simulink model "sldemo_msfcn_edge_detect"  (Simulink 7.6)
settings: Solver=ode45  StartTime=0.0  StopTime=inf  RelTol=1e-3
settings Model: Creator=The MathWorks Inc.  ExtModeAutoUpdateStatusClock=off
settings DataIOCC: SignalLoggingName=logsOut
settings OptimizationCC: InlineInvariantSignals=on  InitFltsAndDblsToZero=on
settings DebuggingCC: SaveWithParameterizedLinksMsg=none  SignalResolutionControl=TryResolveAllWithWarning  SolverPrmCheckMsg=none  InheritedTsInSrcMsg=none  MultiTaskDSMMsg=warning  MultiTaskCondExecSysMsg=none
settings HardwareCC: TargetUnknown=on
settings RTWCC: IncludeERTFirstTime=on
settings GRTTargetCC: TargetFcnLib=ansi_tfl_tmw.mat

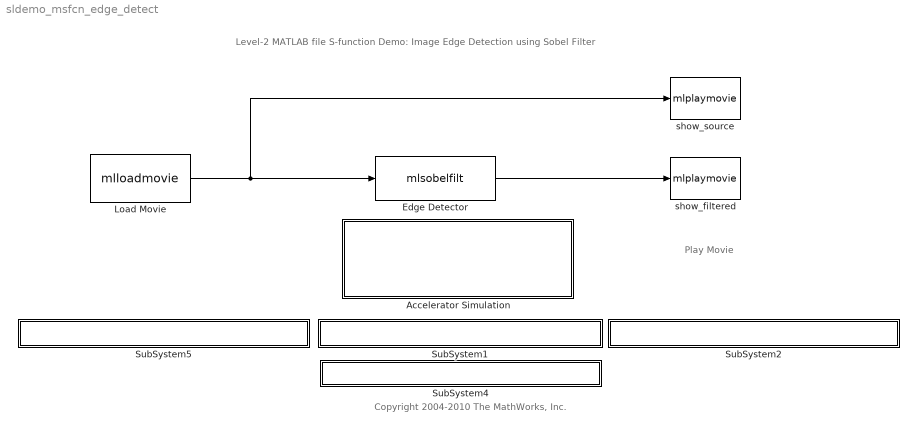
== system sldemo_msfcn_edge_detect ==
  note: Level-2 MATLAB file S-function Demo:
      | Image Edge Detection using Sobel Filter
  note: Play Movie
  note: Copyright 2004-2010 The MathWorks, Inc.
  Accelerator Simulation : Subsystem
      settings: OpenFcn=|
      | set_param(bdroot,'SimulationMode','accelerator');
      | sim(bdroot);
      mask Display: disp('Double click here to run \nsimulation on accelerator using \nTLC for edge detector block');
  Edge Detector : M-S-Function  FunctionName=mlsobelfilt  Parameters=3
  Load Movie : M-S-Function  FunctionName=mlloadmovie  Parameters='sldemoMovie'
  SubSystem1 : Subsystem  mask{filename=mlsobelfilt.m}
      mask init:
      | x=sfundemo_maskdisp;
      settings: AttributesFormatString=\n  OpenFcn=sfundemo_openfcn
      mask Display: disp(x);
  SubSystem2 : Subsystem  mask{filename=mlplaymovie.m}
      mask init:
      | x=sfundemo_maskdisp;
      settings: AttributesFormatString=\n  OpenFcn=sfundemo_openfcn
      mask Display: disp(x);
  SubSystem4 : Subsystem
      settings: OpenFcn=edit(fullfile(matlabroot,'toolbox','simulink','simdemos','simfeatures','mlsobelfilt.tlc'))
      mask Display: disp('matlabroot\toolbox\simulink\simdemos\simfeatures\mlsobelfilt.tlc');
  SubSystem5 : Subsystem  mask{filename=mlloadmovie.m}
      mask init:
      | x=sfundemo_maskdisp;
      settings: AttributesFormatString=\n  OpenFcn=sfundemo_openfcn
      mask Display: disp(x);
  show_filtered : M-S-Function  FunctionName=mlplaymovie  Parameters=122,'Detected Edges'
  show_source : M-S-Function  FunctionName=mlplaymovie  Parameters=121,'Clean Source Image'
  wires:
  Load Movie/1 -> show_source/1, Edge Detector/1
  Edge Detector/1 -> show_filtered/1

== system sldemo_msfcn_edge_detect/Accelerator Simulation ==

== system sldemo_msfcn_edge_detect/SubSystem1 ==

== system sldemo_msfcn_edge_detect/SubSystem2 ==

== system sldemo_msfcn_edge_detect/SubSystem4 ==

== system sldemo_msfcn_edge_detect/SubSystem5 ==
